simulink model "Three_Phase_Half_Wave_Controlled_Rectifier"  (R2017b)
settings: Solver=VariableStepAuto  StartTime=0.0  StopTime=1.0  MaxStep=1e-4  RelTol=1e-3
libraries: powerlib x17, powerlib_meascontrol x7
settings Model: Creator=DELL  LastModifiedBy=DELL

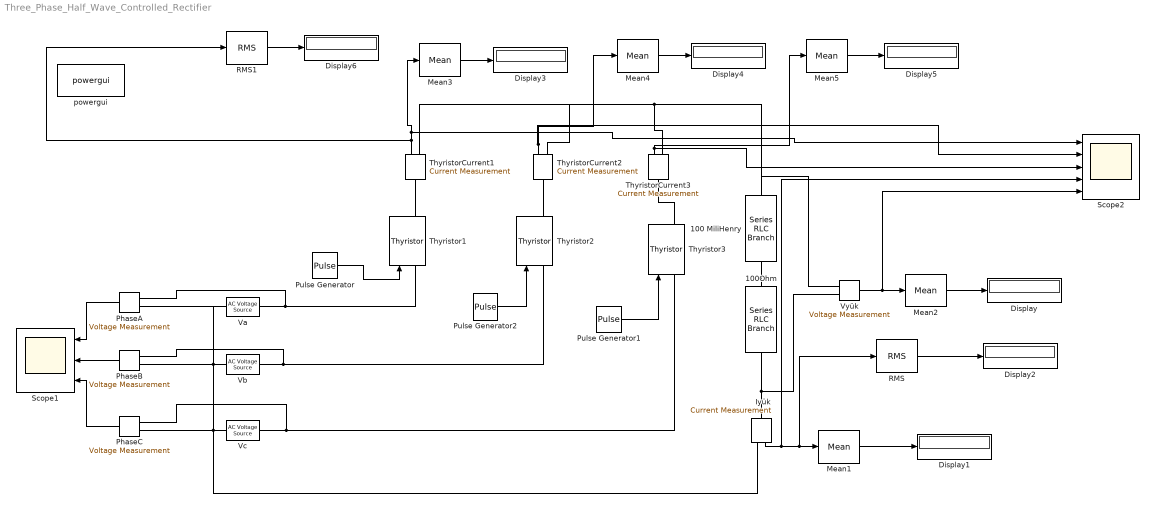
== system Three_Phase_Half_Wave_Controlled_Rectifier ==
  100 MiliHenry : powerlib/Elements/Series RLC Branch  LConnTagsString=__new0  RConnTagsString=__new0  BranchType=L  Resistance=1  Inductance=100e-3  SetiL0=off  InitialCurrent=0  Capacitance=1e-6  Setx0=off  InitialVoltage=0  Measurements=None
  100Ohm : powerlib/Elements/Series RLC Branch  LConnTagsString=__new0  RConnTagsString=__new0  BranchType=R  Resistance=100  Inductance=1e-3  SetiL0=off  InitialCurrent=0  Capacitance=1e-6  Setx0=off  InitialVoltage=0  Measurements=None
  Display{,1..6} (7 alike) : Display
  Iyük : powerlib/Measurements/Current Measurement  PhasorSimulation=off  OutputType=Complex  PSBequivalent=0
  Mean{1..5} (5 alike) : powerlib_meascontrol/Measurements/Mean  Freq=50  Vinit=0  Ts=0
  PhaseA : powerlib/Measurements/Voltage Measurement  PhasorSimulation=off  OutputType=Complex  PSBequivalent=0
  PhaseB : powerlib/Measurements/Voltage Measurement  PhasorSimulation=off  OutputType=Complex  PSBequivalent=0
  PhaseC : powerlib/Measurements/Voltage Measurement  PhasorSimulation=off  OutputType=Complex  PSBequivalent=0
  Pulse Generator : DiscretePulseGenerator  PulseType=Time based  Period=0.02  PulseWidth=5  PhaseDelay=0.01*120/180
  Pulse Generator1 : DiscretePulseGenerator  PulseType=Time based  Period=0.02  PulseWidth=5  PhaseDelay=0.01*360/180
  Pulse Generator2 : DiscretePulseGenerator  PulseType=Time based  Period=0.02  PulseWidth=5  PhaseDelay=0.01*240/180
  RMS : powerlib_meascontrol/Measurements/RMS  TrueRMS=on  Freq=50  RMSInit=120  Ts=0
  RMS1 : powerlib_meascontrol/Measurements/RMS  TrueRMS=on  Freq=50  RMSInit=120  Ts=0
  Scope1 : Scope  NumInputPorts=3
  Scope2 : Scope  NumInputPorts=5
  Thyristor1 : powerlib/Power Electronics/Thyristor  Ron=0.001  Lon=0  Vf=0.8  IC=0  Rs=500  Cs=250e-9  Measurements=on
  Thyristor2 : powerlib/Power Electronics/Thyristor  Ron=0.001  Lon=0  Vf=0.8  IC=0  Rs=500  Cs=250e-9  Measurements=on
  Thyristor3 : powerlib/Power Electronics/Thyristor  Ron=0.001  Lon=0  Vf=0.8  IC=0  Rs=500  Cs=250e-9  Measurements=on
  ThyristorCurrent1 : powerlib/Measurements/Current Measurement  PhasorSimulation=off  OutputType=Complex  PSBequivalent=0
  ThyristorCurrent2 : powerlib/Measurements/Current Measurement  PhasorSimulation=off  OutputType=Complex  PSBequivalent=0
  ThyristorCurrent3 : powerlib/Measurements/Current Measurement  PhasorSimulation=off  OutputType=Complex  PSBequivalent=0
  Va : powerlib/Electrical Sources/AC Voltage Source  Amplitude=220*(2^0.5)  Phase=0  Frequency=50  SampleTime=0  Measurements=None  BusType=swing  Pref=10e3  Qref=0  Qmin=-inf  Qmax=+inf
  Vb : powerlib/Electrical Sources/AC Voltage Source  Amplitude=220*(2^0.5)  Phase=-120  Frequency=50  SampleTime=0  Measurements=None  BusType=swing  Pref=10e3  Qref=0  Qmin=-inf  Qmax=+inf
  Vc : powerlib/Electrical Sources/AC Voltage Source  Amplitude=220*(2^0.5)  Phase=120  Frequency=50  SampleTime=0  Measurements=None  BusType=swing  Pref=10e3  Qref=0  Qmin=-inf  Qmax=+inf
  Vyük : powerlib/Measurements/Voltage Measurement  PhasorSimulation=off  OutputType=Complex  PSBequivalent=0
  powergui : powerlib/powergui  Priority=1  SimulationMode=Continuous  SampleTime=50e-6  frequency=60  Iterations=50  frequencyindice=50  Pbase=100e6  ErrMax=1e-4  UnitsV=kV  UnitsW=MW  buscounter=0  FunctionMessages=off  echomessages=off  EnableUseOfTLC=off  CurrentSourceSwitches=off  DisableSnubberDevices=off  DisableRonSwitches=off  DisableVfSwitches=off  DisplayEquations=off  SolverType=Tustin/Backward Euler (TBE)  Interpol=off  ExternalGateDelay=off  methode=off  Ts=100  x0status=blocks  SPID=on  SwTol=0  HookPort=off  RestoreLinks=warning  ResistiveCurrentMeasurement=off  Frange=[0:2:500]  Ylog=off  Xlog=on  ShowGrid=off  save=off  variable=ZData  structure=0  ZoomFFT=off  StartTime=0.0  cycles=1  DisplayStyle=1  fundamental=60  FreqAxis=off  MaxFrequency=1000  frequencyindicesteady=1  RmsSteady=1  display=off
  wires:
  PhaseB/1 -> Scope1/2
  ThyristorCurrent3/1 -> Scope2/3, Mean5/1
  PhaseC/1 -> Scope1/3
  ThyristorCurrent1/1 -> RMS1/1, Scope2/1, Mean3/1
  Vyük/1 -> Scope2/5, Mean2/1
  Mean2/1 -> Display/1
  Mean1/1 -> Display1/1
  PhaseA/1 -> Scope1/1
  RMS/1 -> Display2/1
  Iyük/1 -> Scope2/4, RMS/1, Mean1/1
  ThyristorCurrent2/1 -> Scope2/2, Mean4/1
  Mean3/1 -> Display3/1
  Mean4/1 -> Display4/1
  Mean5/1 -> Display5/1
  Pulse Generator/1 -> Thyristor1/1
  Pulse Generator1/1 -> Thyristor3/1
  Pulse Generator2/1 -> Thyristor2/1
  RMS1/1 -> Display6/1
  connections:
  Vc/LConn1 -- Iyük/RConn1 -- PhaseC/LConn2 -- Va/LConn1 -- PhaseA/LConn2 -- PhaseB/LConn2 -- Vb/LConn1
  ThyristorCurrent3/RConn1 -- 100 MiliHenry/LConn1 -- Vyük/LConn1 -- ThyristorCurrent1/RConn1 -- ThyristorCurrent2/RConn1
  Vc/RConn1 -- Thyristor3/LConn1 -- PhaseC/LConn1
  Vyük/LConn2 -- Iyük/LConn1 -- 100Ohm/RConn1
  Va/RConn1 -- Thyristor1/LConn1 -- PhaseA/LConn1
  Vb/RConn1 -- Thyristor2/LConn1 -- PhaseB/LConn1
  ThyristorCurrent3/LConn1 -- Thyristor3/RConn1
  Thyristor2/RConn1 -- ThyristorCurrent2/LConn1
  ThyristorCurrent1/LConn1 -- Thyristor1/RConn1
  100Ohm/LConn1 -- 100 MiliHenry/RConn1
